simulink library "VIS_LIB"  (Simulink 8.6)
settings: Solver=ode45  StartTime=0.0  StopTime=10.0  RelTol=1e-3
undefined symbols (not defined in the file): AC, SIXOSEM_F_WD_AC_MASTER
libraries: cdsFilt x376, cdsEpicsOut x253, cdsEpicsIn x179, cdsTP x123, VIS_LIB x95, cdsMuxMatrix x91, cdsEpicsStringIn x75, cdsFiltCtrl x72, cdsFunctionCall x70, cdsRms x59, KAGRA_UTIL x25, STATE_BIO_MASTER x5
(part 21 of 38)

== system VIS_LIB/PReQua_6DOF/DOF_SEL ==
  AMP_LEN : Inport
  AMP_TRA : Inport  Port=2
  AMP_VER : Inport  Port=3
  AMP_ROL : Inport  Port=4
  AMP_PIT : Inport  Port=5
  AMP_YAW : Inport  Port=6
  Phase_LEN : Inport  Port=7
  PHASE_TRA : Inport  Port=8
  PHASE_VER : Inport  Port=9
  PHASE_ROL : Inport  Port=10
  PHASE_PIT : Inport  Port=11
  PHASE_YAW : Inport  Port=12
  FREQ_LEN : Inport  Port=13
  FREQ_TRA : Inport  Port=14
  FREQ_VER : Inport  Port=15
  FREQ_ROL : Inport  Port=16
  FREQ_PIT : Inport  Port=17
  FREQ_YAW : Inport  Port=18
  Q_LEN : Inport  Port=19
  Q_TRA : Inport  Port=20
  Q_VER : Inport  Port=21
  Q_ROL : Inport  Port=22
  Q_PIT : Inport  Port=23
  Q_YAW : Inport  Port=24
  tau_LEN : Inport  Port=25
  tau_TRA : Inport  Port=26
  tau_VER : Inport  Port=27
  tau_ROL : Inport  Port=28
  tau_PIT : Inport  Port=29
  tau_YAW : Inport  Port=30
  AMP : cdsMuxMatrix/Subsystem  Tag=cdsMuxMatrix  Description=Any size matrix. Inputs and outputs must be connected using Mux and Demux parts.
      settings: AttributesFormatString=%<Tag>
  DECAY_TIME : cdsMuxMatrix/Subsystem  Tag=cdsMuxMatrix  Description=Any size matrix. Inputs and outputs must be connected using Mux and Demux parts.
      settings: AttributesFormatString=%<Tag>
  Demux{,1..4} (5 alike) : Demux  Outputs=1
  FREQ : cdsMuxMatrix/Subsystem  Tag=cdsMuxMatrix  Description=Any size matrix. Inputs and outputs must be connected using Mux and Demux parts.
      settings: AttributesFormatString=%<Tag>
  Mux{,1..4} (5 alike) : Mux  Inputs=6
  Q_VAL : cdsMuxMatrix/Subsystem  Tag=cdsMuxMatrix  Description=Any size matrix. Inputs and outputs must be connected using Mux and Demux parts.
      settings: AttributesFormatString=%<Tag>
  REF_PHASE : cdsMuxMatrix/Subsystem  Tag=cdsMuxMatrix  Description=Any size matrix. Inputs and outputs must be connected using Mux and Demux parts.
      settings: AttributesFormatString=%<Tag>
  Sum{,1..5} (6 alike) : Sum  Inputs=-+
  amplitude : Outport
  phase : Outport  Port=2
  RELphase_LEN : Outport  Port=3
  RELphase_TRA : Outport  Port=4
  RELphase_VER : Outport  Port=5
  RELphase_ROL : Outport  Port=6
  RELphase_PIT : Outport  Port=7
  RELphase_YAW : Outport  Port=8
  freq : Outport  Port=9
  q_val : Outport  Port=10
  tau : Outport  Port=11
  wires:
  Demux4/1 -> tau/1
  tau_VER/1 -> Mux4/3
  tau_TRA/1 -> Mux4/2
  tau_PIT/1 -> Mux4/5
  tau_YAW/1 -> Mux4/6
  DECAY_TIME/1 -> Demux4/1
  Mux4/1 -> DECAY_TIME/1
  tau_ROL/1 -> Mux4/4
  tau_LEN/1 -> Mux4/1
  Demux3/1 -> q_val/1
  Q_VER/1 -> Mux3/3
  Q_TRA/1 -> Mux3/2
  Q_PIT/1 -> Mux3/5
  Q_YAW/1 -> Mux3/6
  Q_VAL/1 -> Demux3/1
  Mux3/1 -> Q_VAL/1
  Q_ROL/1 -> Mux3/4
  Q_LEN/1 -> Mux3/1
  Demux2/1 -> freq/1
  FREQ_VER/1 -> Mux2/3
  FREQ_TRA/1 -> Mux2/2
  FREQ_PIT/1 -> Mux2/5
  FREQ_YAW/1 -> Mux2/6
  FREQ/1 -> Demux2/1
  Mux2/1 -> FREQ/1
  FREQ_ROL/1 -> Mux2/4
  FREQ_LEN/1 -> Mux2/1
  Sum/1 -> RELphase_LEN/1
  Sum5/1 -> RELphase_YAW/1
  Sum4/1 -> RELphase_PIT/1
  Sum2/1 -> RELphase_VER/1
  Sum3/1 -> RELphase_ROL/1
  Sum1/1 -> RELphase_TRA/1
  PHASE_YAW/1 -> Sum5/2, Mux1/6
  PHASE_PIT/1 -> Sum4/2, Mux1/5
  PHASE_VER/1 -> Sum2/2, Mux1/3
  PHASE_ROL/1 -> Sum3/2, Mux1/4
  PHASE_TRA/1 -> Sum1/2, Mux1/2
  [REFPHASE] -> Sum/1, Sum1/1, Sum2/1, Sum3/1, Sum4/1, Sum5/1
  Phase_LEN/1 -> Sum/2, Mux1/1
  AMP_VER/1 -> Mux/3
  AMP_TRA/1 -> Mux/2
  REF_PHASE/1 -> Demux1/1
  Mux1/1 -> REF_PHASE/1
  Demux1/1 -> [REFPHASE], phase/1
  Demux/1 -> amplitude/1
  AMP_PIT/1 -> Mux/5
  AMP_YAW/1 -> Mux/6
  AMP/1 -> Demux/1
  Mux/1 -> AMP/1
  AMP_ROL/1 -> Mux/4
  AMP_LEN/1 -> Mux/1

== system VIS_LIB/PReQua_6DOF/normalize ==
  In1 : Inport
  In2 : Inport  Port=2
  In3 : Inport  Port=3
  In4 : Inport  Port=4
  In5 : Inport  Port=5
  In6 : Inport  Port=6
  Divide{,1..5} (6 alike) : Product  Inputs=*/
  Product{,1..5} (6 alike) : Product  RndMeth=Zero
  SQRT : cdsSqrt/Subsystem  Tag=cdsSqrt
      settings: AttributesFormatString=%<Tag>
  Sum : Sum  Inputs=++++++
  Out1 : Outport
  Out2 : Outport  Port=2
  Out3 : Outport  Port=3
  Out4 : Outport  Port=4
  Out5 : Outport  Port=5
  Out6 : Outport  Port=6
  wires:
  Divide5/1 -> Out6/1
  Divide4/1 -> Out5/1
  Divide3/1 -> Out4/1
  Divide2/1 -> Out3/1
  Divide1/1 -> Out2/1
  Divide/1 -> Out1/1
  [NORM] -> Divide/2, Divide1/2, Divide2/2, Divide3/2, Divide4/2, Divide5/2
  In2/1 -> Product1/2, Product1/1, Divide1/1
  Product4/1 -> Sum/5
  Product2/1 -> Sum/3
  Product/1 -> Sum/1
  Product5/1 -> Sum/6
  Product3/1 -> Sum/4
  Sum/1 -> SQRT/1
  In1/1 -> Product/2, Product/1, Divide/1
  Product1/1 -> Sum/2
  In5/1 -> Product4/2, Product4/1, Divide4/1
  In4/1 -> Product3/2, Product3/1, Divide3/1
  In3/1 -> Product2/2, Product2/1, Divide2/1
  SQRT/1 -> [NORM]
  In6/1 -> Product5/2, Product5/1, Divide5/1

== system VIS_LIB/QUAASC1/CP_COEF ==
  note: #DAQ Channels
      |
      | ITM_PIT_OUT 128
      | ETM_PIT_OUT 128
      | ITM_YAW_OUT 128
      | ETM_YAW_OUT 128
  LEN_IN : Inport
  TRA_IN : Inport  Port=2
  VER_IN : Inport  Port=3
  ROL_IN : Inport  Port=4
  ETM_PIT : cdsFilt/Subsystem  Tag=cdsFilt  Description=|
      | Purpose:                                                                                                                                                                                                                                  
      | Standard CDS IIR filter module.                                                                                                                                                                                                           
      |                                                                                                                                                                                                                                           
      | Operation:                                                                                                                                                                                                                                
      | Consists of 10 second order section IIR filters, plus a ramped gain stage. In FE code, also provides pre-defined test points and excitation channel inputs. The filter coefficients are defined in the LIGO system using the 'foton' tool.
      |                                                                                                                                                                                                                                           
      | Usage:                                                                                                                                                                                                                                    
      | Name the part with the desired filter module name.
      settings: AttributesFormatString=%<Tag>
  ETM_YAW : cdsFilt/Subsystem  Tag=cdsFilt  Description=|
      | Purpose:                                                                                                                                                                                                                                  
      | Standard CDS IIR filter module.                                                                                                                                                                                                           
      |                                                                                                                                                                                                                                           
      | Operation:                                                                                                                                                                                                                                
      | Consists of 10 second order section IIR filters, plus a ramped gain stage. In FE code, also provides pre-defined test points and excitation channel inputs. The filter coefficients are defined in the LIGO system using the 'foton' tool.
      |                                                                                                                                                                                                                                           
      | Usage:                                                                                                                                                                                                                                    
      | Name the part with the desired filter module name.
      settings: AttributesFormatString=%<Tag>
  ITM_PIT : cdsFilt/Subsystem  Tag=cdsFilt  Description=|
      | Purpose:                                                                                                                                                                                                                                  
      | Standard CDS IIR filter module.                                                                                                                                                                                                           
      |                                                                                                                                                                                                                                           
      | Operation:                                                                                                                                                                                                                                
      | Consists of 10 second order section IIR filters, plus a ramped gain stage. In FE code, also provides pre-defined test points and excitation channel inputs. The filter coefficients are defined in the LIGO system using the 'foton' tool.
      |                                                                                                                                                                                                                                           
      | Usage:                                                                                                                                                                                                                                    
      | Name the part with the desired filter module name.
      settings: AttributesFormatString=%<Tag>
  ITM_YAW : cdsFilt/Subsystem  Tag=cdsFilt  Description=|
      | Purpose:                                                                                                                                                                                                                                  
      | Standard CDS IIR filter module.                                                                                                                                                                                                           
      |                                                                                                                                                                                                                                           
      | Operation:                                                                                                                                                                                                                                
      | Consists of 10 second order section IIR filters, plus a ramped gain stage. In FE code, also provides pre-defined test points and excitation channel inputs. The filter coefficients are defined in the LIGO system using the 'foton' tool.
      |                                                                                                                                                                                                                                           
      | Usage:                                                                                                                                                                                                                                    
      | Name the part with the desired filter module name.
      settings: AttributesFormatString=%<Tag>
  LEN_OUT : Outport
  TRA_OUT : Outport  Port=2
  VER_OUT : Outport  Port=3
  ROL_OUT : Outport  Port=4
  wires:
  ETM_PIT/1 -> VER_OUT/1
  VER_IN/1 -> ETM_PIT/1
  TRA_IN/1 -> ITM_YAW/1
  ITM_YAW/1 -> TRA_OUT/1
  ETM_YAW/1 -> ROL_OUT/1
  ROL_IN/1 -> ETM_YAW/1
  LEN_IN/1 -> ITM_PIT/1
  ITM_PIT/1 -> LEN_OUT/1

== system VIS_LIB/QUAASC1/DOF_SEL ==
  Phase_LEN : Inport
  PHASE_TRA : Inport  Port=2
  PHASE_VER : Inport  Port=3
  PHASE_ROL : Inport  Port=4
  Demux1 : Demux  Outputs=1
  Mux1 : Mux
  REF_PHASE : cdsMuxMatrix/Subsystem  Tag=cdsMuxMatrix  Description=Any size matrix. Inputs and outputs must be connected using Mux and Demux parts.
      settings: AttributesFormatString=%<Tag>
  Sum{,1..3} (4 alike) : Sum  Inputs=-+
  RELphase_LEN : Outport
  RELphase_TRA : Outport  Port=2
  RELphase_VER : Outport  Port=3
  RELphase_ROL : Outport  Port=4
  wires:
  Sum/1 -> RELphase_LEN/1
  Sum2/1 -> RELphase_VER/1
  Sum3/1 -> RELphase_ROL/1
  Sum1/1 -> RELphase_TRA/1
  PHASE_VER/1 -> Sum2/2, Mux1/3
  PHASE_ROL/1 -> Sum3/2, Mux1/4
  PHASE_TRA/1 -> Sum1/2, Mux1/2
  [REFPHASE] -> Sum/1, Sum1/1, Sum2/1, Sum3/1
  Phase_LEN/1 -> Sum/2, Mux1/1
  REF_PHASE/1 -> Demux1/1
  Mux1/1 -> REF_PHASE/1
  Demux1/1 -> [REFPHASE]

== system VIS_LIB/QUAASC1/REL_PHASE ==
  note: #DAQ Channels
      |
      | ITM_PIT_OUT 128
      | ETM_PIT_OUT 128
      | ITM_YAW_OUT 128
      | ETM_YAW_OUT 128
  LEN_IN : Inport
  TRA_IN : Inport  Port=2
  VER_IN : Inport  Port=3
  ROL_IN : Inport  Port=4
  ETM_PIT : cdsFilt/Subsystem  Tag=cdsFilt  Description=|
      | Purpose:                                                                                                                                                                                                                                  
      | Standard CDS IIR filter module.                                                                                                                                                                                                           
      |                                                                                                                                                                                                                                           
      | Operation:                                                                                                                                                                                                                                
      | Consists of 10 second order section IIR filters, plus a ramped gain stage. In FE code, also provides pre-defined test points and excitation channel inputs. The filter coefficients are defined in the LIGO system using the 'foton' tool.
      |                                                                                                                                                                                                                                           
      | Usage:                                                                                                                                                                                                                                    
      | Name the part with the desired filter module name.
      settings: AttributesFormatString=%<Tag>
  ETM_YAW : cdsFilt/Subsystem  Tag=cdsFilt  Description=|
      | Purpose:                                                                                                                                                                                                                                  
      | Standard CDS IIR filter module.                                                                                                                                                                                                           
      |                                                                                                                                                                                                                                           
      | Operation:                                                                                                                                                                                                                                
      | Consists of 10 second order section IIR filters, plus a ramped gain stage. In FE code, also provides pre-defined test points and excitation channel inputs. The filter coefficients are defined in the LIGO system using the 'foton' tool.
      |                                                                                                                                                                                                                                           
      | Usage:                                                                                                                                                                                                                                    
      | Name the part with the desired filter module name.
      settings: AttributesFormatString=%<Tag>
  ITM_PIT : cdsFilt/Subsystem  Tag=cdsFilt  Description=|
      | Purpose:                                                                                                                                                                                                                                  
      | Standard CDS IIR filter module.                                                                                                                                                                                                           
      |                                                                                                                                                                                                                                           
      | Operation:                                                                                                                                                                                                                                
      | Consists of 10 second order section IIR filters, plus a ramped gain stage. In FE code, also provides pre-defined test points and excitation channel inputs. The filter coefficients are defined in the LIGO system using the 'foton' tool.
      |                                                                                                                                                                                                                                           
      | Usage:                                                                                                                                                                                                                                    
      | Name the part with the desired filter module name.
      settings: AttributesFormatString=%<Tag>
  ITM_YAW : cdsFilt/Subsystem  Tag=cdsFilt  Description=|
      | Purpose:                                                                                                                                                                                                                                  
      | Standard CDS IIR filter module.                                                                                                                                                                                                           
      |                                                                                                                                                                                                                                           
      | Operation:                                                                                                                                                                                                                                
      | Consists of 10 second order section IIR filters, plus a ramped gain stage. In FE code, also provides pre-defined test points and excitation channel inputs. The filter coefficients are defined in the LIGO system using the 'foton' tool.
      |                                                                                                                                                                                                                                           
      | Usage:                                                                                                                                                                                                                                    
      | Name the part with the desired filter module name.
      settings: AttributesFormatString=%<Tag>
  LEN_OUT : Outport
  TRA_OUT : Outport  Port=2
  VER_OUT : Outport  Port=3
  ROL_OUT : Outport  Port=4
  wires:
  ITM_PIT/1 -> LEN_OUT/1
  LEN_IN/1 -> ITM_PIT/1
  ROL_IN/1 -> ETM_YAW/1
  ETM_YAW/1 -> ROL_OUT/1
  ITM_YAW/1 -> TRA_OUT/1
  TRA_IN/1 -> ITM_YAW/1
  VER_IN/1 -> ETM_PIT/1
  ETM_PIT/1 -> VER_OUT/1

== system VIS_LIB/QUAASC1/normalize ==
  In1 : Inport
  In2 : Inport  Port=2
  In3 : Inport  Port=3
  In4 : Inport  Port=4
  Divide{,1..3} (4 alike) : Product  Inputs=*/
  Product{,1..3} (4 alike) : Product  RndMeth=Zero
  SQRT : cdsSqrt/Subsystem  Tag=cdsSqrt
      settings: AttributesFormatString=%<Tag>
  Sum : Sum  Inputs=++++
  Out1 : Outport
  Out2 : Outport  Port=2
  Out3 : Outport  Port=3
  Out4 : Outport  Port=4
  wires:
  Divide3/1 -> Out4/1
  Divide2/1 -> Out3/1
  Divide1/1 -> Out2/1
  Divide/1 -> Out1/1
  [NORM] -> Divide/2, Divide1/2, Divide2/2, Divide3/2
  In2/1 -> Product1/2, Product1/1, Divide1/1
  Product2/1 -> Sum/3
  Product/1 -> Sum/1
  Product3/1 -> Sum/4
  Sum/1 -> SQRT/1
  In1/1 -> Product/2, Product/1, Divide/1
  Product1/1 -> Sum/2
  In4/1 -> Product3/2, Product3/1, Divide3/1
  In3/1 -> Product2/2, Product2/1, Divide2/1
  SQRT/1 -> [NORM]

== system VIS_LIB/UTILs/1COIL_DQ ==
  note: #DAQ Channels
      |
      | GAS_OUT 256
  iGAS : Inport
  GAS : cdsFilt/Subsystem  Tag=cdsFilt  Description=|
      | Purpose:                                                                                                                                                                                                                                  
      | Standard CDS IIR filter module.                                                                                                                                                                                                           
      |                                                                                                                                                                                                                                           
      | Operation:                                                                                                                                                                                                                                
      | Consists of 10 second order section IIR filters, plus a ramped gain stage. In FE code, also provides pre-defined test points and excitation channel inputs. The filter coefficients are defined in the LIGO system using the 'foton' tool.
      |                                                                                                                                                                                                                                           
      | Usage:                                                                                                                                                                                                                                    
      | Name the part with the desired filter module name.
      settings: AttributesFormatString=%<Tag>
  oGAS : Outport
  wires:
  iGAS/1 -> GAS/1
  GAS/1 -> oGAS/1

== system VIS_LIB/UTILs/3COILs ==
  iH1 : Inport
  iH2 : Inport  Port=2
  iH3 : Inport  Port=3
  H1 : cdsFilt/Subsystem  Tag=cdsFilt  Description=|
      | Purpose:                                                                                                                                                                                                                                  
      | Standard CDS IIR filter module.                                                                                                                                                                                                           
      |                                                                                                                                                                                                                                           
      | Operation:                                                                                                                                                                                                                                
      | Consists of 10 second order section IIR filters, plus a ramped gain stage. In FE code, also provides pre-defined test points and excitation channel inputs. The filter coefficients are defined in the LIGO system using the 'foton' tool.
      |                                                                                                                                                                                                                                           
      | Usage:                                                                                                                                                                                                                                    
      | Name the part with the desired filter module name.
      settings: AttributesFormatString=%<Tag>
  H2 : cdsFilt/Subsystem  Tag=cdsFilt  Description=|
      | Purpose:                                                                                                                                                                                                                                  
      | Standard CDS IIR filter module.                                                                                                                                                                                                           
      |                                                                                                                                                                                                                                           
      | Operation:                                                                                                                                                                                                                                
      | Consists of 10 second order section IIR filters, plus a ramped gain stage. In FE code, also provides pre-defined test points and excitation channel inputs. The filter coefficients are defined in the LIGO system using the 'foton' tool.
      |                                                                                                                                                                                                                                           
      | Usage:                                                                                                                                                                                                                                    
      | Name the part with the desired filter module name.
      settings: AttributesFormatString=%<Tag>
  H3 : cdsFilt/Subsystem  Tag=cdsFilt  Description=|
      | Purpose:                                                                                                                                                                                                                                  
      | Standard CDS IIR filter module.                                                                                                                                                                                                           
      |                                                                                                                                                                                                                                           
      | Operation:                                                                                                                                                                                                                                
      | Consists of 10 second order section IIR filters, plus a ramped gain stage. In FE code, also provides pre-defined test points and excitation channel inputs. The filter coefficients are defined in the LIGO system using the 'foton' tool.
      |                                                                                                                                                                                                                                           
      | Usage:                                                                                                                                                                                                                                    
      | Name the part with the desired filter module name.
      settings: AttributesFormatString=%<Tag>
  oH1 : Outport
  oH2 : Outport  Port=2
  oH3 : Outport  Port=3
  wires:
  iH3/1 -> H3/1
  H3/1 -> oH3/1
  iH2/1 -> H2/1
  H2/1 -> oH2/1
  iH1/1 -> H1/1
  H1/1 -> oH1/1

== system VIS_LIB/UTILs/3COILs_DQ ==
  note: #DAQ Channels
      |
      | H1_OUT 256
      | H2_OUT 256
      | H3_OUT 256
  iH1 : Inport
  iH2 : Inport  Port=2
  iH3 : Inport  Port=3
  H1 : cdsFilt/Subsystem  Tag=cdsFilt  Description=|
      | Purpose:                                                                                                                                                                                                                                  
      | Standard CDS IIR filter module.                                                                                                                                                                                                           
      |                                                                                                                                                                                                                                           
      | Operation:                                                                                                                                                                                                                                
      | Consists of 10 second order section IIR filters, plus a ramped gain stage. In FE code, also provides pre-defined test points and excitation channel inputs. The filter coefficients are defined in the LIGO system using the 'foton' tool.
      |                                                                                                                                                                                                                                           
      | Usage:                                                                                                                                                                                                                                    
      | Name the part with the desired filter module name.
      settings: AttributesFormatString=%<Tag>
  H2 : cdsFilt/Subsystem  Tag=cdsFilt  Description=|
      | Purpose:                                                                                                                                                                                                                                  
      | Standard CDS IIR filter module.                                                                                                                                                                                                           
      |                                                                                                                                                                                                                                           
      | Operation:                                                                                                                                                                                                                                
      | Consists of 10 second order section IIR filters, plus a ramped gain stage. In FE code, also provides pre-defined test points and excitation channel inputs. The filter coefficients are defined in the LIGO system using the 'foton' tool.
      |                                                                                                                                                                                                                                           
      | Usage:                                                                                                                                                                                                                                    
      | Name the part with the desired filter module name.
      settings: AttributesFormatString=%<Tag>
  H3 : cdsFilt/Subsystem  Tag=cdsFilt  Description=|
      | Purpose:                                                                                                                                                                                                                                  
      | Standard CDS IIR filter module.                                                                                                                                                                                                           
      |                                                                                                                                                                                                                                           
      | Operation:                                                                                                                                                                                                                                
      | Consists of 10 second order section IIR filters, plus a ramped gain stage. In FE code, also provides pre-defined test points and excitation channel inputs. The filter coefficients are defined in the LIGO system using the 'foton' tool.
      |                                                                                                                                                                                                                                           
      | Usage:                                                                                                                                                                                                                                    
      | Name the part with the desired filter module name.
      settings: AttributesFormatString=%<Tag>
  oH1 : Outport
  oH2 : Outport  Port=2
  oH3 : Outport  Port=3
  wires:
  iH3/1 -> H3/1
  H3/1 -> oH3/1
  iH2/1 -> H2/1
  H2/1 -> oH2/1
  iH1/1 -> H1/1
  H1/1 -> oH1/1

== system VIS_LIB/UTILs/4COILs ==
  iH1 : Inport
  iH2 : Inport  Port=2
  iH3 : Inport  Port=3
  iH4 : Inport  Port=4
  H1 : cdsFilt/Subsystem  Tag=cdsFilt  Description=|
      | Purpose:                                                                                                                                                                                                                                  
      | Standard CDS IIR filter module.                                                                                                                                                                                                           
      |                                                                                                                                                                                                                                           
      | Operation:                                                                                                                                                                                                                                
      | Consists of 10 second order section IIR filters, plus a ramped gain stage. In FE code, also provides pre-defined test points and excitation channel inputs. The filter coefficients are defined in the LIGO system using the 'foton' tool.
      |                                                                                                                                                                                                                                           
      | Usage:                                                                                                                                                                                                                                    
      | Name the part with the desired filter module name.
      settings: AttributesFormatString=%<Tag>
  H2 : cdsFilt/Subsystem  Tag=cdsFilt  Description=|
      | Purpose:                                                                                                                                                                                                                                  
      | Standard CDS IIR filter module.                                                                                                                                                                                                           
      |                                                                                                                                                                                                                                           
      | Operation:                                                                                                                                                                                                                                
      | Consists of 10 second order section IIR filters, plus a ramped gain stage. In FE code, also provides pre-defined test points and excitation channel inputs. The filter coefficients are defined in the LIGO system using the 'foton' tool.
      |                                                                                                                                                                                                                                           
      | Usage:                                                                                                                                                                                                                                    
      | Name the part with the desired filter module name.
      settings: AttributesFormatString=%<Tag>
  H3 : cdsFilt/Subsystem  Tag=cdsFilt  Description=|
      | Purpose:                                                                                                                                                                                                                                  
      | Standard CDS IIR filter module.                                                                                                                                                                                                           
      |                                                                                                                                                                                                                                           
      | Operation:                                                                                                                                                                                                                                
      | Consists of 10 second order section IIR filters, plus a ramped gain stage. In FE code, also provides pre-defined test points and excitation channel inputs. The filter coefficients are defined in the LIGO system using the 'foton' tool.
      |                                                                                                                                                                                                                                           
      | Usage:                                                                                                                                                                                                                                    
      | Name the part with the desired filter module name.
      settings: AttributesFormatString=%<Tag>
  H4 : cdsFilt/Subsystem  Tag=cdsFilt  Description=|
      | Purpose:                                                                                                                                                                                                                                  
      | Standard CDS IIR filter module.                                                                                                                                                                                                           
      |                                                                                                                                                                                                                                           
      | Operation:                                                                                                                                                                                                                                
      | Consists of 10 second order section IIR filters, plus a ramped gain stage. In FE code, also provides pre-defined test points and excitation channel inputs. The filter coefficients are defined in the LIGO system using the 'foton' tool.
      |                                                                                                                                                                                                                                           
      | Usage:                                                                                                                                                                                                                                    
      | Name the part with the desired filter module name.
      settings: AttributesFormatString=%<Tag>
  oH1 : Outport
  oH2 : Outport  Port=2
  oH3 : Outport  Port=3
  oH4 : Outport  Port=4
  wires:
  H1/1 -> oH1/1
  iH1/1 -> H1/1
  H2/1 -> oH2/1
  iH2/1 -> H2/1
  H3/1 -> oH3/1
  iH3/1 -> H3/1
  iH4/1 -> H4/1
  H4/1 -> oH4/1
